simulink model "TSCLAB_ModelByte_11"  (R2021a)
settings: Solver=VariableStepAuto  StartTime=0.0  StopTime=600  RelTol=1e-3
libraries: instrumentseriallib x3
settings Model: Creator=vasanza  LastModifiedBy=vasan
settings SolverCC: AlgebraicLoopSolver=TrustRegion
settings DebuggingCC: SFMachineParentedDataDiag=warning

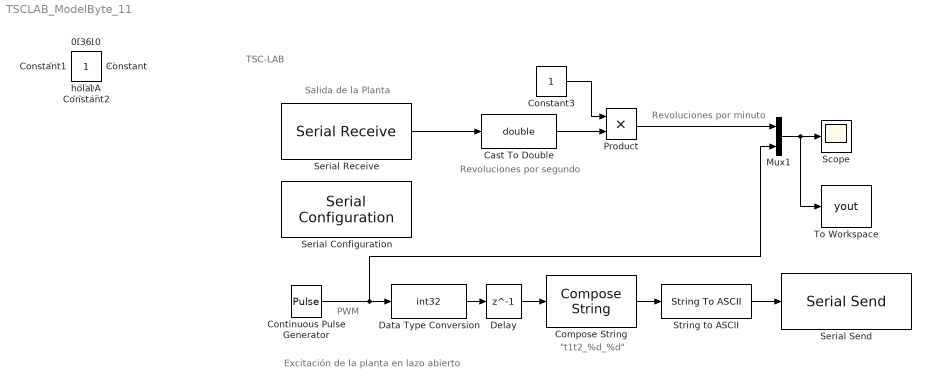
== system TSCLAB_ModelByte_11 ==
  note: "t1t2_%d_%d"
  note: PWM
  note: Excitación de la planta en lazo abierto
  note: Revoluciones por minuto
  note: Revoluciones por segundo
  note: Salida de la Planta
  note: TSC-LAB
  Cast To Double : DataTypeConversion  OutDataTypeStr=double
  Compose String : ComposeString  Format="\"t1_%d\""
  Constant3 : Constant
  Continuous Pulse Generator : DiscretePulseGenerator  PulseType=Time based  Amplitude=255  Period=600  PulseWidth=50
  Data Type Conversion : DataTypeConversion  OutDataTypeStr=int32
  Delay : Delay  DelayLength=1  InitialCondition=0
  Mux1 : Mux  Inputs=2
  Product : Product
  Scope : Scope
  Serial Configuration : instrumentseriallib/Serial Configuration  Priority=-200000  Port=<Select a port...>  ComPort=<Select a port...>  BaudRate=115200  DataBits=8  Parity=none  StopBits=1  ByteOrder=little-endian  FlowControl=none  Timeout=10  SimulateUsing=Interpreted execution  BlockInModel=on
  Serial Receive : instrumentseriallib/Serial Receive  Port=<Select a port...>  ComPort=<Select a port...>  DataType=uint8  SaveDataType=uint8  ToggleHeader=off  Header=[]  ToggleTerminator=on  Terminator=<none>  CustomTerminator=[]  ToggleDataSize=on  DataSize=[1 1]  EnableBlockingMode=on  ActionDataUnavailable=Output last received value  ActionWhenDataUnavailable=Output last received value  CustomValue=0  SampleTime=0.999  SimulateUsing=Interpreted execution  BlockInModel=on
  Serial Send : instrumentseriallib/Serial Send  Port=<Select a port...>  ComPort=<Select a port...>  Header=[]  Terminator=<none>  CustomTerminator=[]  EnableBlockingMode=on  SimulateUsing=Interpreted execution  BlockInModel=on
  String to ASCII : StringToASCII
  To Workspace : ToWorkspace  VariableName=yout  SampleTime=-1
      settings: Save2DSignal=2-D array (concatenate along first dimension)
  $ : Constant  IOType=siggen  Value=36
  , : Constant  IOType=siggen  Value=44
  {0,10,255,311,12345} (5 alike) : Constant  IOType=siggen
  0A : Constant  IOType=siggen  Value=10
  0D : Constant  IOType=siggen  Value=13
  13 : Constant  IOType=siggen  Value=13
  36 : Constant  IOType=siggen  Value=36
  Constant : Constant  IOType=siggen
  Constant1 : Constant  IOType=siggen
  Constant2 : Constant  IOType=siggen
  hola : Constant  IOType=siggen
  wires:
  Mux1/1 -> To Workspace/1, Scope/1
  Data Type Conversion/1 -> Delay/1
  Serial Receive/1 -> Cast To Double/1
  Cast To Double/1 -> Product/2
  Constant3/1 -> Product/1
  Product/1 -> Mux1/1
  Delay/1 -> Compose String/1
  Compose String/1 -> String to ASCII/1
  String to ASCII/1 -> Serial Send/1
  Continuous Pulse Generator/1 -> Data Type Conversion/1, Mux1/2
